simulink model "simulinkProject"  (R2023a)
settings: Solver=ode4  StartTime=0.0  StopTime=20  FixedStep=System.Ts  RelTol=1e-3
values from neighbouring files (symbols this model uses):
  b_end = 0.5*(K_end * (Lift.m + Tilt.m + Cylinder_3.m + Extension_2.m + Extension_1.m + Cylinder_4.m))^0.5    [project.m]
  b_end_1 = 0.5*(K_end_1 * (Lift.m + Pillar.m + Cylinder.m + Tilt.m + Cylinder_4.m + Cylinder_3.m + Extension_1.m + Extension_2.m))^0.5    [project.m]
  b_end_3 = 0.5*(K_end_3 * (Tilt.m + Extension_2.m + Extension_1.m + Cylinder_4.m))^0.5    [project.m]
  b_end_4 = 0.5*(K_end_4 * (Extension_2.m + Extension_1.m))^0.5    [project.m]
  K_end = p_max / delta_x    [project.m]
  K_end_1 = p_max_1 / delta_x_1    [project.m]
  K_end_3 = p_max_3 / delta_x_3    [project.m]
  K_end_4 = p_max_4 / delta_x_4    [project.m]
  Offset = 0.92    [project.m]
  Offset_1 = 0.72    [project.m]
  Offset_4 = 2.640    (= 2.64)    [project.m]
undefined symbols (not defined in the file or in its folder): Cylinder, Cylinder_1, Cylinder_3, Cylinder_4, Extension_1, fabs, Fourbar_1, Fourbar_2, Lift, Pillar, Pinion, Piston, Piston_3, Piston_4, sgn, System, System_1, System_3, System_4, Tilt, Valve, Valve_1, Valve_3, Valve_4, X, Y, Z
libraries: sm_lib x71, nesl_utility x27, TcTargetLib x1
(part 1 of 4)
settings Model: Creator=aless  LastModifiedBy=aless
settings OptimizationCC: DefaultParameterBehavior=Inlined  LocalBlockOutputs=off
settings RTWCC: Description=TwinCAT GRT Target  SystemTargetFile=TwinCatGrt.tlc  GenCodeOnly=on  GenerateMakefile=off  TemplateMakefile=tcgrt_msbuild.tmf  TargetLang=C++
settings STFCustomTargetCC: TargetLangStandard=C++11 (ISO)  CombineOutputUpdateFcns=on  CodeInterfacePackaging=Reusable function  CPPClassGenCompliant=on  GRTInterface=off  GenerateAllocFcn=on  UseToolchainInfoCompliant=off  SystemTargetFile=TwinCatGrt.tlc
settings GRTTargetCC: TargetLangStandard=C++11 (ISO)  ParMdlRefBuildCompliant=off  CompOptLevelCompliant=off  MatFileLogging=off  CodeInterfacePackaging=Reusable function  GenerateAllocFcn=on  UseToolchainInfoCompliant=off  ExtModeMexFile=TcExtModeClient

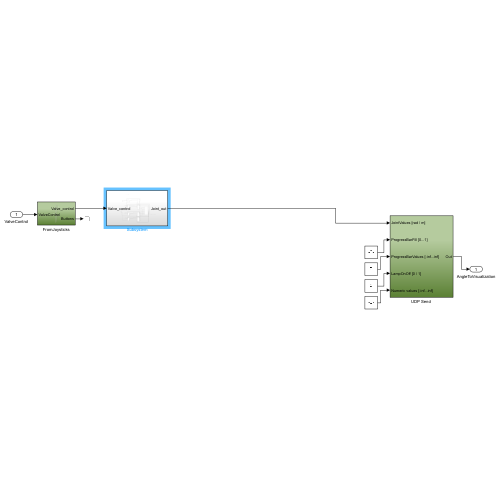
[thumbnail: Simulink's stored preview of the top-level diagram]
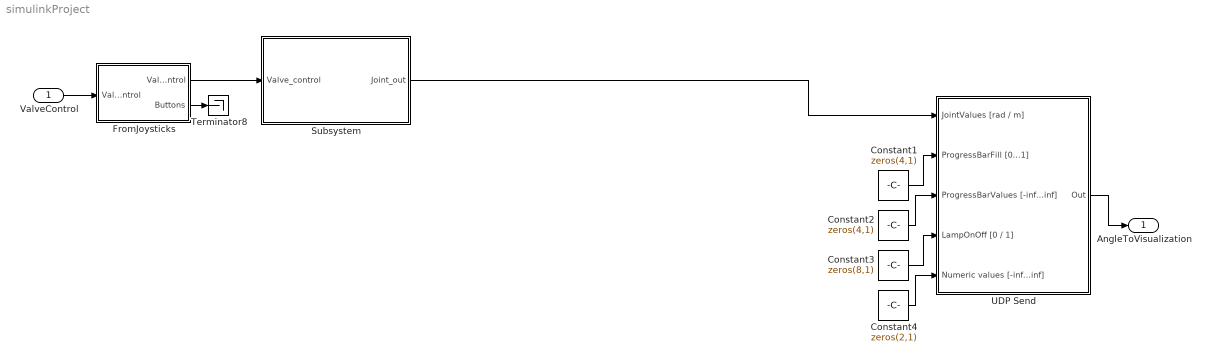
== system simulinkProject ==
  ValveControl : Inport  OutDataTypeStr=double  PortDimensions=19
  Constant1 : Constant  Value=zeros(4,1)
  Constant2 : Constant  Value=zeros(4,1)
  Constant3 : Constant  Value=zeros(8,1)
  Constant4 : Constant  Value=zeros(2,1)
  FromJoysticks : Subsystem
  Subsystem : Subsystem
  Terminator8 : Terminator
  "UDP Send " : Subsystem
  AngleToVisualization : Outport  OutDataTypeStr=single  PortDimensions=22
  wires:
  FromJoysticks/2(Buttons) -> Terminator8/1
  FromJoysticks/1(Valve_control) -> Subsystem/1(Valve_control)
  ValveControl/1 -> FromJoysticks/1(ValveControl)
  "UDP Send "/1(Out) -> AngleToVisualization/1
  Constant2/1 -> "UDP Send "/3(ProgressBarValues [-inf...inf])
  Subsystem/1(Joint_out) -> "UDP Send "/1(JointValues [rad / m])
  Constant1/1 -> "UDP Send "/2(ProgressBarFill [0...1])
  Constant3/1 -> "UDP Send "/4(LampOnOff [0 / 1])
  Constant4/1 -> "UDP Send "/5(Numeric values [-inf...inf])

== system simulinkProject/FromJoysticks ==
  ValveControl : Inport  OutDataTypeStr=double  PortDimensions=19
  Demux : Demux  Outputs=19
  Mux : Mux
  Mux1 : Mux  Inputs=15
  Valve_control : Outport
  Buttons : Outport  Port=2
  wires:
  ValveControl/1 -> Demux/1
  Demux/13 -> Mux1/9
  Demux/15 -> Mux1/11
  Demux/12 -> Mux1/8
  Demux/3 -> Mux/3
  Demux/11 -> Mux1/7
  Demux/16 -> Mux1/12
  Demux/14 -> Mux1/10
  Mux/1 -> Valve_control/1
  Demux/1 -> Mux/1
  Demux/9 -> Mux1/5
  Mux1/1 -> Buttons/1
  Demux/4 -> Mux/4
  Demux/6 -> Mux1/2
  Demux/2 -> Mux/2
  Demux/7 -> Mux1/3
  Demux/10 -> Mux1/6
  Demux/5 -> Mux1/1
  Demux/8 -> Mux1/4
  Demux/17 -> Mux1/13
  Demux/18 -> Mux1/14
  Demux/19 -> Mux1/15

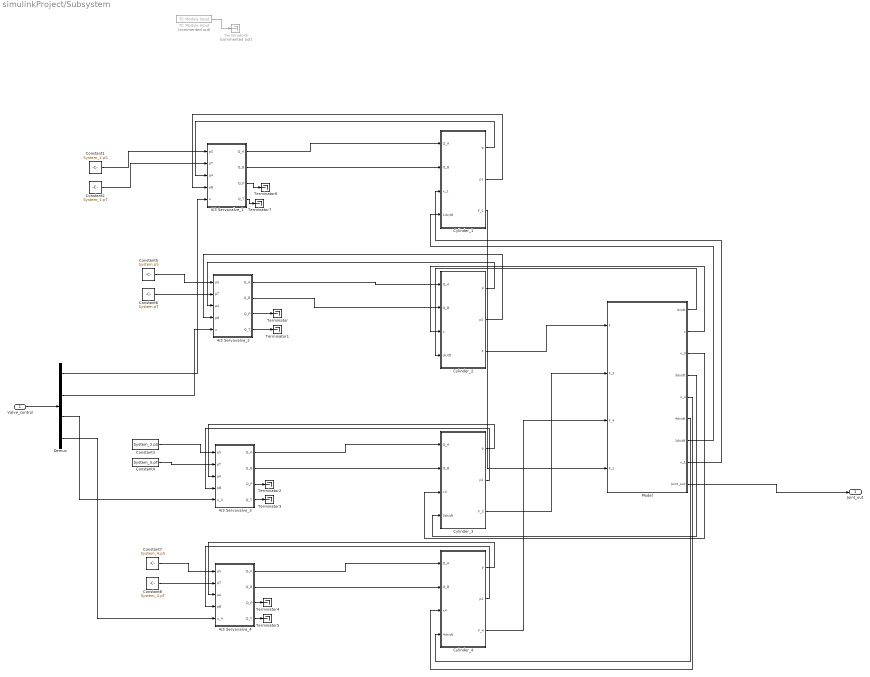
== system simulinkProject/Subsystem ==
  Valve_control : Inport
  4/3 Servovalve_1 : Subsystem  mask(Hydraulic){QN=Valve_1.QN, dpN=Valve_1.dpN, ptr=Valve_1.ptr}
      mask prompts: QN "Nominal flow [m^3/s] :"; dpN "Nominal pressure difference per notch [Pa] :"; ptr "Transition Pressure [Pa] :"
  4/3 Servovalve_2 : Subsystem  mask(Hydraulic){QN=Valve.QN, dpN=Valve.dpN, ptr=Valve.ptr}
      mask prompts: QN "Nominal flow [m^3/s] :"; dpN "Nominal pressure difference per notch [Pa] :"; ptr "Transition Pressure [Pa] :"
  4/3 Servovalve_3 : Subsystem  mask(Hydraulic){QN=Valve_3.QN, dpN=Valve_3.dpN, ptr=Valve_3.ptr}
      mask prompts: QN "Nominal flow [m^3/s] :"; dpN "Nominal pressure difference per notch [Pa] :"; ptr "Transition Pressure [Pa] :"
  4/3 Servovalve_4 : Subsystem  mask(Hydraulic){QN=Valve_4.QN, dpN=Valve_4.dpN, ptr=Valve_4.ptr}
      mask prompts: QN "Nominal flow [m^3/s] :"; dpN "Nominal pressure difference per notch [Pa] :"; ptr "Transition Pressure [Pa] :"
  Constant1 : Constant  Value=System_1.pS
  Constant2 : Constant  Value=System_1.pT
  Constant3 : Constant  Value=System_3.pS
  Constant4 : Constant  Value=System_3.pT
  Constant5 : Constant  Value=System.pS
  Constant6 : Constant  Value=System.pT
  Constant7 : Constant  Value=System_4.pS
  Constant8 : Constant  Value=System_4.pT
  Cylinder_1 : Subsystem
  Cylinder_2 : Subsystem
  Cylinder_3 : Subsystem
  Cylinder_4 : Subsystem
  Demux : Demux
  Model : Subsystem
  TC Module Input : TcTargetLib/TC Module Input  Commented=on  PortDataType=double  PortDim=1  Value=0  SampleTime=-1  CodeGenConnectType=DataArea (InputDst)  DataTypeOverride=off
  Terminator{,1..7} (8 alike) : Terminator
  Terminator8 : Terminator  Commented=on
  Joint_out : Outport
  wires:
  Cylinder_1/3(F_1) -> Model/4(F_1)
  Cylinder_2/1(p) -> 4/3 Servovalve_2/3(pA)
  Model/2(x) -> Cylinder_2/3(x)
  Constant7/1 -> 4/3 Servovalve_4/1(pS)
  Model/8(x_1) -> Cylinder_1/3(x_1)
  4/3 Servovalve_2/2(Q_B) -> Cylinder_2/2(Q_B)
  4/3 Servovalve_1/3(Q_P) -> Terminator6/1
  4/3 Servovalve_2/3(Q_P) -> Terminator/1
  4/3 Servovalve_4/1(Q_A) -> Cylinder_4/1(Q_A)
  Cylinder_4/2(p1) -> 4/3 Servovalve_4/4(pB)
  Cylinder_2/3(F) -> Model/1(F)
  4/3 Servovalve_2/4(Q_T) -> Terminator1/1
  Model/6(4dx/dt) -> Cylinder_4/4(4dx/dt)
  4/3 Servovalve_3/4(Q_T) -> Terminator3/1
  Cylinder_3/2(p1) -> 4/3 Servovalve_3/4(pB)
  Cylinder_4/3(F_4) -> Model/3(F_4)
  Model/5(x_4) -> Cylinder_4/3(x4)
  4/3 Servovalve_3/1(Q_A) -> Cylinder_3/1(Q_A)
  Demux/1 -> 4/3 Servovalve_1/5(u)
  Cylinder_3/3(F_3) -> Model/2(F_3)
  Constant2/1 -> 4/3 Servovalve_1/2(pT)
  Constant3/1 -> 4/3 Servovalve_3/1(pS)
  4/3 Servovalve_2/1(Q_A) -> Cylinder_2/1(Q_A)
  Model/9(Joint_out) -> Joint_out/1
  Cylinder_2/2(p1) -> 4/3 Servovalve_2/4(pB)
  4/3 Servovalve_3/2(Q_B) -> Cylinder_3/2(Q_B)
  Model/3(x_3) -> Cylinder_3/3(x3)
  Cylinder_3/1(p) -> 4/3 Servovalve_3/3(pA)
  4/3 Servovalve_4/2(Q_B) -> Cylinder_4/2(Q_B)
  Model/1(dx/dt) -> Cylinder_2/4(dx/dt)
  4/3 Servovalve_4/4(Q_T) -> Terminator5/1
  Constant4/1 -> 4/3 Servovalve_3/2(pT)
  Model/4(3dx/dt) -> Cylinder_3/4(3dx/dt)
  Constant6/1 -> 4/3 Servovalve_2/2(pT)
  4/3 Servovalve_1/1(Q_A) -> Cylinder_1/1(Q_A)
  Cylinder_4/1(p) -> 4/3 Servovalve_4/3(pA)
  Constant1/1 -> 4/3 Servovalve_1/1(pS)
  4/3 Servovalve_4/3(Q_P) -> Terminator4/1
  4/3 Servovalve_1/4(Q_T) -> Terminator7/1
  Constant5/1 -> 4/3 Servovalve_2/1(pS)
  Demux/2 -> 4/3 Servovalve_2/5(u)
  Constant8/1 -> 4/3 Servovalve_4/2(pT)
  4/3 Servovalve_1/2(Q_B) -> Cylinder_1/2(Q_B)
  4/3 Servovalve_3/3(Q_P) -> Terminator2/1
  Valve_control/1 -> Demux/1
  Cylinder_1/1(p) -> 4/3 Servovalve_1/3(pA)
  Model/7(1dx/dt) -> Cylinder_1/4(1dx/dt)
  Cylinder_1/2(p1) -> 4/3 Servovalve_1/4(pB)
  Demux/4 -> 4/3 Servovalve_4/5(u_4)
  TC Module Input/1 -> Terminator8/1
  Demux/3 -> 4/3 Servovalve_3/5(u_3)

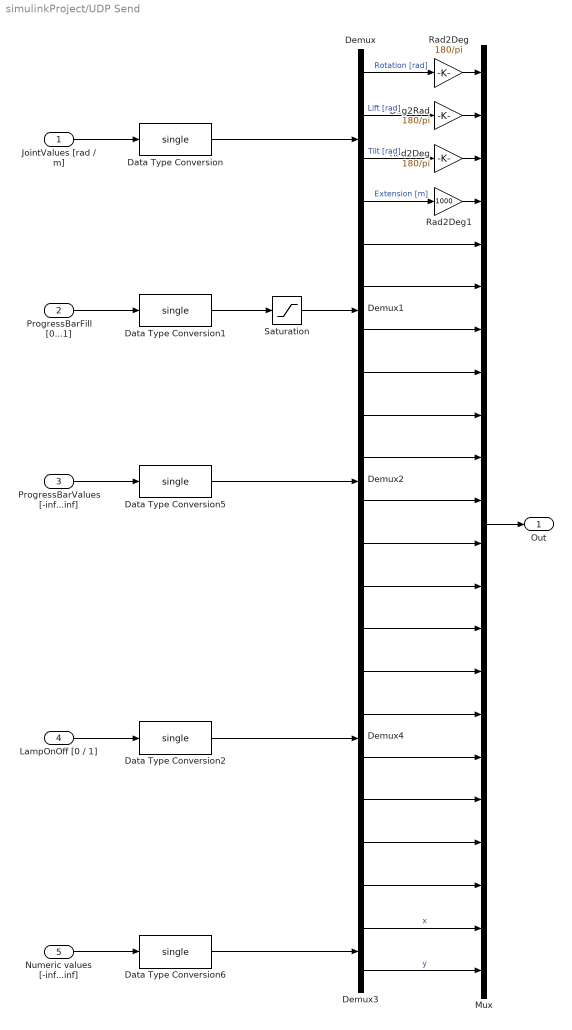
== system simulinkProject/UDP Send  ==
  JointValues [rad / m] : Inport
  ProgressBarFill [0...1] : Inport  Port=2
  ProgressBarValues [-inf...inf] : Inport  Port=3
  LampOnOff [0 / 1] : Inport  Port=4
  Numeric values [-inf...inf] : Inport  Port=5
  Data Type Conversion{,1..2,5..6} (5 alike) : DataTypeConversion  OutDataTypeStr=single  SaturateOnIntegerOverflow=off  RndMeth=Floor
  "Deg2Rad " : Gain  Gain=180/pi
  Demux : Demux
  Demux1 : Demux
  Demux2 : Demux
  Demux3 : Demux  Outputs=2
  Demux4 : Demux  Outputs=8
  Mux : Mux  Inputs=22
  Rad2Deg : Gain  Gain=180/pi
  "Rad2Deg " : Gain  Gain=180/pi
  Rad2Deg1 : Gain  Gain=1000
  Saturation : Saturate  UpperLimit=1  LowerLimit=0
  Out : Outport  OutDataTypeStr=single  PortDimensions=22
  wires:
  JointValues [rad / m]/1 -> Data Type Conversion/1
  Demux/4 -> Rad2Deg1/1  "Extension [m]"
  Demux/2 -> "Deg2Rad "/1  "Lift [rad]"
  Demux/3 -> Rad2Deg/1  "Tilt [rad]"
  Demux/1 -> "Rad2Deg "/1  "Rotation [rad]"
  "Rad2Deg "/1 -> Mux/1
  "Deg2Rad "/1 -> Mux/2
  Rad2Deg/1 -> Mux/3
  Data Type Conversion/1 -> Demux/1
  Demux1/1 -> Mux/5
  Demux1/2 -> Mux/6
  Demux1/3 -> Mux/7
  Demux1/4 -> Mux/8
  Demux2/1 -> Mux/9
  Demux2/2 -> Mux/10
  Demux2/3 -> Mux/11
  Demux2/4 -> Mux/12
  Data Type Conversion1/1 -> Saturation/1
  Data Type Conversion5/1 -> Demux2/1
  Demux4/1 -> Mux/13
  Demux4/2 -> Mux/14
  Demux4/3 -> Mux/15
  Demux4/4 -> Mux/16
  Demux4/5 -> Mux/17
  Demux4/6 -> Mux/18
  Demux4/7 -> Mux/19
  Demux4/8 -> Mux/20
  Demux3/1 -> Mux/21  "x"
  Demux3/2 -> Mux/22  "y"
  LampOnOff [0 / 1]/1 -> Data Type Conversion2/1
  Data Type Conversion2/1 -> Demux4/1
  Saturation/1 -> Demux1/1
  ProgressBarFill [0...1]/1 -> Data Type Conversion1/1
  ProgressBarValues [-inf...inf]/1 -> Data Type Conversion5/1
  Numeric values [-inf...inf]/1 -> Data Type Conversion6/1
  Data Type Conversion6/1 -> Demux3/1
  Mux/1 -> Out/1
  Rad2Deg1/1 -> Mux/4

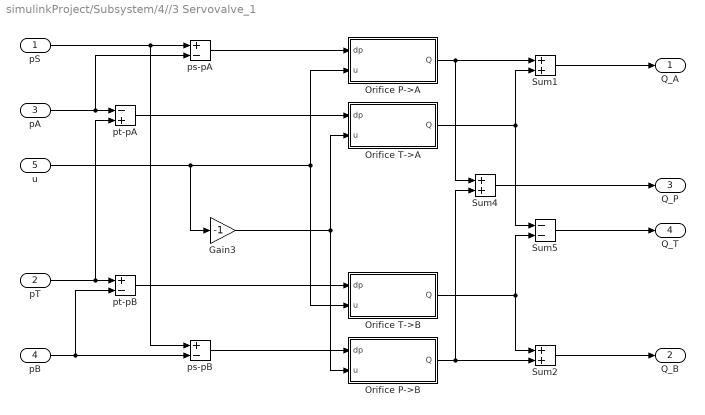
== system simulinkProject/Subsystem/4//3 Servovalve_1 ==
  pS : Inport
  pT : Inport  Port=2
  pA : Inport  Port=3
  pB : Inport  Port=4
  u : Inport  Port=5
  Gain3 : Gain  Gain=-1  SaturateOnIntegerOverflow=on  OutDataTypeStr=Inherit: Same as input  ParamDataTypeStr=Inherit: Same as input
  Orifice P->A : Subsystem  mask(Hydraulic){QN=QN, AN=1, DPN=dpN, ptr=ptr}
      mask prompts: QN "Nominal Flow [m^3/s] :"; AN "Nominal opening [ 0...1 ] :"; DPN "Nominal Pressure Difference [Pa] :"; ptr "Transition Pressure [Pa] :"
      mask help:
      | Implements numerically robust turbulent flow
      | equation. Polynomial flow equation is used
      | when abs(dp) < Transition Pressure.
      mask init:
      | K = QN/(AN*sqrt(DPN));
      mask Help: eval('hydlibdoc(''orificedoc'')')
  Orifice P->B : Subsystem  mask(Hydraulic){QN=QN, AN=1, DPN=dpN, ptr=ptr}
      mask prompts: QN "Nominal Flow [m^3/s] :"; AN "Nominal opening [ 0...1 ] :"; DPN "Nominal Pressure Difference [Pa] :"; ptr "Transition Pressure [Pa] :"
      mask help:
      | Implements numerically robust turbulent flow
      | equation. Polynomial flow equation is used
      | when abs(dp) < Transition Pressure.
      mask init:
      | K = QN/(AN*sqrt(DPN));
      mask Help: eval('hydlibdoc(''orificedoc'')')
  Orifice T->A : Subsystem  mask(Hydraulic){QN=QN, AN=1, DPN=dpN, ptr=ptr}
      mask prompts: QN "Nominal Flow [m^3/s] :"; AN "Nominal opening [ 0...1 ] :"; DPN "Nominal Pressure Difference [Pa] :"; ptr "Transition Pressure [Pa] :"
      mask help:
      | Implements numerically robust turbulent flow
      | equation. Polynomial flow equation is used
      | when abs(dp) < Transition Pressure.
      mask init:
      | K = QN/(AN*sqrt(DPN));
      mask Help: eval('hydlibdoc(''orificedoc'')')
  Orifice T->B : Subsystem  mask(Hydraulic){QN=QN, AN=1, DPN=dpN, ptr=ptr}
      mask prompts: QN "Nominal Flow [m^3/s] :"; AN "Nominal opening [ 0...1 ] :"; DPN "Nominal Pressure Difference [Pa] :"; ptr "Transition Pressure [Pa] :"
      mask help:
      | Implements numerically robust turbulent flow
      | equation. Polynomial flow equation is used
      | when abs(dp) < Transition Pressure.
      mask init:
      | K = QN/(AN*sqrt(DPN));
      mask Help: eval('hydlibdoc(''orificedoc'')')
  Sum1 : Sum  InputSameDT=on  SaturateOnIntegerOverflow=on  OutDataTypeStr=Inherit: Same as first input
  Sum2 : Sum  InputSameDT=on  SaturateOnIntegerOverflow=on  OutDataTypeStr=Inherit: Same as first input
  Sum4 : Sum  InputSameDT=on  SaturateOnIntegerOverflow=on  OutDataTypeStr=Inherit: Same as first input
  Sum5 : Sum  Inputs=--  InputSameDT=on  SaturateOnIntegerOverflow=on  OutDataTypeStr=Inherit: Same as first input
  ps-pA : Sum  Inputs=+-  InputSameDT=on  SaturateOnIntegerOverflow=on  OutDataTypeStr=Inherit: Same as first input
  ps-pB : Sum  Inputs=+-  InputSameDT=on  SaturateOnIntegerOverflow=on  OutDataTypeStr=Inherit: Same as first input
  pt-pA : Sum  Inputs=-+  InputSameDT=on  SaturateOnIntegerOverflow=on  OutDataTypeStr=Inherit: Same as first input
  pt-pB : Sum  Inputs=+-  InputSameDT=on  SaturateOnIntegerOverflow=on  OutDataTypeStr=Inherit: Same as first input
  Q_A : Outport  VectorParamsAs1DForOutWhenUnconnected=off
  Q_B : Outport  Port=2  VectorParamsAs1DForOutWhenUnconnected=off
  Q_P : Outport  Port=3  VectorParamsAs1DForOutWhenUnconnected=off
  Q_T : Outport  Port=4  VectorParamsAs1DForOutWhenUnconnected=off
  wires:
  Gain3/1 -> Orifice P->B/2(u), Orifice T->A/2(u)
  pt-pB/1 -> Orifice T->B/1(dp)
  ps-pB/1 -> Orifice P->B/1(dp)
  ps-pA/1 -> Orifice P->A/1(dp)
  pt-pA/1 -> Orifice T->A/1(dp)
  Sum5/1 -> Q_T/1
  Sum4/1 -> Q_P/1
  Orifice P->A/1(Q) -> Sum4/1, Sum1/1
  Orifice P->B/1(Q) -> Sum4/2, Sum2/2
  u/1 -> Orifice T->B/2(u), Orifice P->A/2(u), Gain3/1
  pB/1 -> pt-pB/2, ps-pB/2
  Orifice T->B/1(Q) -> Sum2/1, Sum5/2
  Sum2/1 -> Q_B/1
  pT/1 -> pt-pA/2, pt-pB/1
  pA/1 -> ps-pA/2, pt-pA/1
  pS/1 -> ps-pA/1, ps-pB/1
  Orifice T->A/1(Q) -> Sum1/2, Sum5/1
  Sum1/1 -> Q_A/1

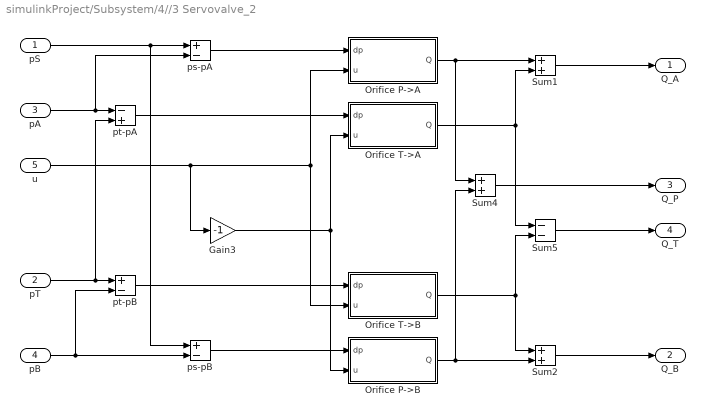
== system simulinkProject/Subsystem/4//3 Servovalve_2 ==
  pS : Inport
  pT : Inport  Port=2
  pA : Inport  Port=3
  pB : Inport  Port=4
  u : Inport  Port=5
  Gain3 : Gain  Gain=-1  SaturateOnIntegerOverflow=on  OutDataTypeStr=Inherit: Same as input  ParamDataTypeStr=Inherit: Same as input
  Orifice P->A : Subsystem  mask(Hydraulic){QN=QN, AN=1, DPN=dpN, ptr=ptr}
      mask prompts: QN "Nominal Flow [m^3/s] :"; AN "Nominal opening [ 0...1 ] :"; DPN "Nominal Pressure Difference [Pa] :"; ptr "Transition Pressure [Pa] :"
      mask help:
      | Implements numerically robust turbulent flow
      | equation. Polynomial flow equation is used
      | when abs(dp) < Transition Pressure.
      mask init:
      | K = QN/(AN*sqrt(DPN));
      mask Help: eval('hydlibdoc(''orificedoc'')')
  Orifice P->B : Subsystem  mask(Hydraulic){QN=QN, AN=1, DPN=dpN, ptr=ptr}
      mask prompts: QN "Nominal Flow [m^3/s] :"; AN "Nominal opening [ 0...1 ] :"; DPN "Nominal Pressure Difference [Pa] :"; ptr "Transition Pressure [Pa] :"
      mask help:
      | Implements numerically robust turbulent flow
      | equation. Polynomial flow equation is used
      | when abs(dp) < Transition Pressure.
      mask init:
      | K = QN/(AN*sqrt(DPN));
      mask Help: eval('hydlibdoc(''orificedoc'')')
  Orifice T->A : Subsystem  mask(Hydraulic){QN=QN, AN=1, DPN=dpN, ptr=ptr}
      mask prompts: QN "Nominal Flow [m^3/s] :"; AN "Nominal opening [ 0...1 ] :"; DPN "Nominal Pressure Difference [Pa] :"; ptr "Transition Pressure [Pa] :"
      mask help:
      | Implements numerically robust turbulent flow
      | equation. Polynomial flow equation is used
      | when abs(dp) < Transition Pressure.
      mask init:
      | K = QN/(AN*sqrt(DPN));
      mask Help: eval('hydlibdoc(''orificedoc'')')
  Orifice T->B : Subsystem  mask(Hydraulic){QN=QN, AN=1, DPN=dpN, ptr=ptr}
      mask prompts: QN "Nominal Flow [m^3/s] :"; AN "Nominal opening [ 0...1 ] :"; DPN "Nominal Pressure Difference [Pa] :"; ptr "Transition Pressure [Pa] :"
      mask help:
      | Implements numerically robust turbulent flow
      | equation. Polynomial flow equation is used
      | when abs(dp) < Transition Pressure.
      mask init:
      | K = QN/(AN*sqrt(DPN));
      mask Help: eval('hydlibdoc(''orificedoc'')')
  Sum1 : Sum  InputSameDT=on  SaturateOnIntegerOverflow=on  OutDataTypeStr=Inherit: Same as first input
  Sum2 : Sum  InputSameDT=on  SaturateOnIntegerOverflow=on  OutDataTypeStr=Inherit: Same as first input
  Sum4 : Sum  InputSameDT=on  SaturateOnIntegerOverflow=on  OutDataTypeStr=Inherit: Same as first input
  Sum5 : Sum  Inputs=--  InputSameDT=on  SaturateOnIntegerOverflow=on  OutDataTypeStr=Inherit: Same as first input
  ps-pA : Sum  Inputs=+-  InputSameDT=on  SaturateOnIntegerOverflow=on  OutDataTypeStr=Inherit: Same as first input
  ps-pB : Sum  Inputs=+-  InputSameDT=on  SaturateOnIntegerOverflow=on  OutDataTypeStr=Inherit: Same as first input
  pt-pA : Sum  Inputs=-+  InputSameDT=on  SaturateOnIntegerOverflow=on  OutDataTypeStr=Inherit: Same as first input
  pt-pB : Sum  Inputs=+-  InputSameDT=on  SaturateOnIntegerOverflow=on  OutDataTypeStr=Inherit: Same as first input
  Q_A : Outport  VectorParamsAs1DForOutWhenUnconnected=off
  Q_B : Outport  Port=2  VectorParamsAs1DForOutWhenUnconnected=off
  Q_P : Outport  Port=3  VectorParamsAs1DForOutWhenUnconnected=off
  Q_T : Outport  Port=4  VectorParamsAs1DForOutWhenUnconnected=off
  wires:
  Gain3/1 -> Orifice P->B/2(u), Orifice T->A/2(u)
  pt-pB/1 -> Orifice T->B/1(dp)
  ps-pB/1 -> Orifice P->B/1(dp)
  ps-pA/1 -> Orifice P->A/1(dp)
  pt-pA/1 -> Orifice T->A/1(dp)
  Sum5/1 -> Q_T/1
  Sum4/1 -> Q_P/1
  Orifice P->A/1(Q) -> Sum4/1, Sum1/1
  Orifice P->B/1(Q) -> Sum4/2, Sum2/2
  u/1 -> Orifice T->B/2(u), Orifice P->A/2(u), Gain3/1
  pB/1 -> pt-pB/2, ps-pB/2
  Orifice T->B/1(Q) -> Sum2/1, Sum5/2
  Sum2/1 -> Q_B/1
  pT/1 -> pt-pA/2, pt-pB/1
  pA/1 -> ps-pA/2, pt-pA/1
  pS/1 -> ps-pA/1, ps-pB/1
  Orifice T->A/1(Q) -> Sum1/2, Sum5/1
  Sum1/1 -> Q_A/1

== system simulinkProject/Subsystem/4//3 Servovalve_3 ==
  pS : Inport
  pT : Inport  Port=2
  pA : Inport  Port=3
  pB : Inport  Port=4
  u_3 : Inport  Port=5
  Gain3 : Gain  Gain=-1  SaturateOnIntegerOverflow=on  OutDataTypeStr=Inherit: Same as input  ParamDataTypeStr=Inherit: Same as input
  Orifice P->A : Subsystem  mask(Hydraulic){QN=QN, AN=1, DPN=dpN, ptr=ptr}
      mask prompts: QN "Nominal Flow [m^3/s] :"; AN "Nominal opening [ 0...1 ] :"; DPN "Nominal Pressure Difference [Pa] :"; ptr "Transition Pressure [Pa] :"
      mask help:
      | Implements numerically robust turbulent flow
      | equation. Polynomial flow equation is used
      | when abs(dp) < Transition Pressure.
      mask init:
      | K = QN/(AN*sqrt(DPN));
      mask Help: eval('hydlibdoc(''orificedoc'')')
  Orifice P->B : Subsystem  mask(Hydraulic){QN=QN, AN=1, DPN=dpN, ptr=ptr}
      mask prompts: QN "Nominal Flow [m^3/s] :"; AN "Nominal opening [ 0...1 ] :"; DPN "Nominal Pressure Difference [Pa] :"; ptr "Transition Pressure [Pa] :"
      mask help:
      | Implements numerically robust turbulent flow
      | equation. Polynomial flow equation is used
      | when abs(dp) < Transition Pressure.
      mask init:
      | K = QN/(AN*sqrt(DPN));
      mask Help: eval('hydlibdoc(''orificedoc'')')
  Orifice T->A : Subsystem  mask(Hydraulic){QN=QN, AN=1, DPN=dpN, ptr=ptr}
      mask prompts: QN "Nominal Flow [m^3/s] :"; AN "Nominal opening [ 0...1 ] :"; DPN "Nominal Pressure Difference [Pa] :"; ptr "Transition Pressure [Pa] :"
      mask help:
      | Implements numerically robust turbulent flow
      | equation. Polynomial flow equation is used
      | when abs(dp) < Transition Pressure.
      mask init:
      | K = QN/(AN*sqrt(DPN));
      mask Help: eval('hydlibdoc(''orificedoc'')')
  Orifice T->B : Subsystem  mask(Hydraulic){QN=QN, AN=1, DPN=dpN, ptr=ptr}
      mask prompts: QN "Nominal Flow [m^3/s] :"; AN "Nominal opening [ 0...1 ] :"; DPN "Nominal Pressure Difference [Pa] :"; ptr "Transition Pressure [Pa] :"
      mask help:
      | Implements numerically robust turbulent flow
      | equation. Polynomial flow equation is used
      | when abs(dp) < Transition Pressure.
      mask init:
      | K = QN/(AN*sqrt(DPN));
      mask Help: eval('hydlibdoc(''orificedoc'')')
  Sum1 : Sum  InputSameDT=on  SaturateOnIntegerOverflow=on  OutDataTypeStr=Inherit: Same as first input
  Sum2 : Sum  InputSameDT=on  SaturateOnIntegerOverflow=on  OutDataTypeStr=Inherit: Same as first input
  Sum4 : Sum  InputSameDT=on  SaturateOnIntegerOverflow=on  OutDataTypeStr=Inherit: Same as first input
  Sum5 : Sum  Inputs=--  InputSameDT=on  SaturateOnIntegerOverflow=on  OutDataTypeStr=Inherit: Same as first input
  ps-pA : Sum  Inputs=+-  InputSameDT=on  SaturateOnIntegerOverflow=on  OutDataTypeStr=Inherit: Same as first input
  ps-pB : Sum  Inputs=+-  InputSameDT=on  SaturateOnIntegerOverflow=on  OutDataTypeStr=Inherit: Same as first input
  pt-pA : Sum  Inputs=-+  InputSameDT=on  SaturateOnIntegerOverflow=on  OutDataTypeStr=Inherit: Same as first input
  pt-pB : Sum  Inputs=+-  InputSameDT=on  SaturateOnIntegerOverflow=on  OutDataTypeStr=Inherit: Same as first input
  Q_A : Outport  VectorParamsAs1DForOutWhenUnconnected=off
  Q_B : Outport  Port=2  VectorParamsAs1DForOutWhenUnconnected=off
  Q_P : Outport  Port=3  VectorParamsAs1DForOutWhenUnconnected=off
  Q_T : Outport  Port=4  VectorParamsAs1DForOutWhenUnconnected=off
  wires:
  Gain3/1 -> Orifice P->B/2(u), Orifice T->A/2(u)
  pt-pB/1 -> Orifice T->B/1(dp)
  ps-pB/1 -> Orifice P->B/1(dp)
  ps-pA/1 -> Orifice P->A/1(dp)
  pt-pA/1 -> Orifice T->A/1(dp)
  Sum5/1 -> Q_T/1
  Sum4/1 -> Q_P/1
  Orifice P->A/1(Q) -> Sum4/1, Sum1/1
  Orifice P->B/1(Q) -> Sum4/2, Sum2/2
  u_3/1 -> Orifice T->B/2(u), Orifice P->A/2(u), Gain3/1
  pB/1 -> pt-pB/2, ps-pB/2
  Orifice T->B/1(Q) -> Sum2/1, Sum5/2
  Sum2/1 -> Q_B/1
  pT/1 -> pt-pA/2, pt-pB/1
  pA/1 -> ps-pA/2, pt-pA/1
  pS/1 -> ps-pA/1, ps-pB/1
  Orifice T->A/1(Q) -> Sum1/2, Sum5/1
  Sum1/1 -> Q_A/1

== system simulinkProject/Subsystem/4//3 Servovalve_4 ==
  pS : Inport
  pT : Inport  Port=2
  pA : Inport  Port=3
  pB : Inport  Port=4
  u_4 : Inport  Port=5
  Gain3 : Gain  Gain=-1  SaturateOnIntegerOverflow=on  OutDataTypeStr=Inherit: Same as input  ParamDataTypeStr=Inherit: Same as input
  Orifice P->A : Subsystem  mask(Hydraulic){QN=QN, AN=1, DPN=dpN, ptr=ptr}
      mask prompts: QN "Nominal Flow [m^3/s] :"; AN "Nominal opening [ 0...1 ] :"; DPN "Nominal Pressure Difference [Pa] :"; ptr "Transition Pressure [Pa] :"
      mask help:
      | Implements numerically robust turbulent flow
      | equation. Polynomial flow equation is used
      | when abs(dp) < Transition Pressure.
      mask init:
      | K = QN/(AN*sqrt(DPN));
      mask Help: eval('hydlibdoc(''orificedoc'')')
  Orifice P->B : Subsystem  mask(Hydraulic){QN=QN, AN=1, DPN=dpN, ptr=ptr}
      mask prompts: QN "Nominal Flow [m^3/s] :"; AN "Nominal opening [ 0...1 ] :"; DPN "Nominal Pressure Difference [Pa] :"; ptr "Transition Pressure [Pa] :"
      mask help:
      | Implements numerically robust turbulent flow
      | equation. Polynomial flow equation is used
      | when abs(dp) < Transition Pressure.
      mask init:
      | K = QN/(AN*sqrt(DPN));
      mask Help: eval('hydlibdoc(''orificedoc'')')
  Orifice T->A : Subsystem  mask(Hydraulic){QN=QN, AN=1, DPN=dpN, ptr=ptr}
      mask prompts: QN "Nominal Flow [m^3/s] :"; AN "Nominal opening [ 0...1 ] :"; DPN "Nominal Pressure Difference [Pa] :"; ptr "Transition Pressure [Pa] :"
      mask help:
      | Implements numerically robust turbulent flow
      | equation. Polynomial flow equation is used
      | when abs(dp) < Transition Pressure.
      mask init:
      | K = QN/(AN*sqrt(DPN));
      mask Help: eval('hydlibdoc(''orificedoc'')')
  Orifice T->B : Subsystem  mask(Hydraulic){QN=QN, AN=1, DPN=dpN, ptr=ptr}
      mask prompts: QN "Nominal Flow [m^3/s] :"; AN "Nominal opening [ 0...1 ] :"; DPN "Nominal Pressure Difference [Pa] :"; ptr "Transition Pressure [Pa] :"
      mask help:
      | Implements numerically robust turbulent flow
      | equation. Polynomial flow equation is used
      | when abs(dp) < Transition Pressure.
      mask init:
      | K = QN/(AN*sqrt(DPN));
      mask Help: eval('hydlibdoc(''orificedoc'')')
  Sum1 : Sum  InputSameDT=on  SaturateOnIntegerOverflow=on  OutDataTypeStr=Inherit: Same as first input
  Sum2 : Sum  InputSameDT=on  SaturateOnIntegerOverflow=on  OutDataTypeStr=Inherit: Same as first input
  Sum4 : Sum  InputSameDT=on  SaturateOnIntegerOverflow=on  OutDataTypeStr=Inherit: Same as first input
  Sum5 : Sum  Inputs=--  InputSameDT=on  SaturateOnIntegerOverflow=on  OutDataTypeStr=Inherit: Same as first input
  ps-pA : Sum  Inputs=+-  InputSameDT=on  SaturateOnIntegerOverflow=on  OutDataTypeStr=Inherit: Same as first input
  ps-pB : Sum  Inputs=+-  InputSameDT=on  SaturateOnIntegerOverflow=on  OutDataTypeStr=Inherit: Same as first input
  pt-pA : Sum  Inputs=-+  InputSameDT=on  SaturateOnIntegerOverflow=on  OutDataTypeStr=Inherit: Same as first input
  pt-pB : Sum  Inputs=+-  InputSameDT=on  SaturateOnIntegerOverflow=on  OutDataTypeStr=Inherit: Same as first input
  Q_A : Outport  VectorParamsAs1DForOutWhenUnconnected=off
  Q_B : Outport  Port=2  VectorParamsAs1DForOutWhenUnconnected=off
  Q_P : Outport  Port=3  VectorParamsAs1DForOutWhenUnconnected=off
  Q_T : Outport  Port=4  VectorParamsAs1DForOutWhenUnconnected=off
  wires:
  Gain3/1 -> Orifice P->B/2(u), Orifice T->A/2(u)
  pt-pB/1 -> Orifice T->B/1(dp)
  ps-pB/1 -> Orifice P->B/1(dp)
  ps-pA/1 -> Orifice P->A/1(dp)
  pt-pA/1 -> Orifice T->A/1(dp)
  Sum5/1 -> Q_T/1
  Sum4/1 -> Q_P/1
  Orifice P->A/1(Q) -> Sum4/1, Sum1/1
  Orifice P->B/1(Q) -> Sum4/2, Sum2/2
  u_4/1 -> Orifice T->B/2(u), Orifice P->A/2(u), Gain3/1
  pB/1 -> pt-pB/2, ps-pB/2
  Orifice T->B/1(Q) -> Sum2/1, Sum5/2
  Sum2/1 -> Q_B/1
  pT/1 -> pt-pA/2, pt-pB/1
  pA/1 -> ps-pA/2, pt-pA/1
  pS/1 -> ps-pA/1, ps-pB/1
  Orifice T->A/1(Q) -> Sum1/2, Sum5/1
  Sum1/1 -> Q_A/1

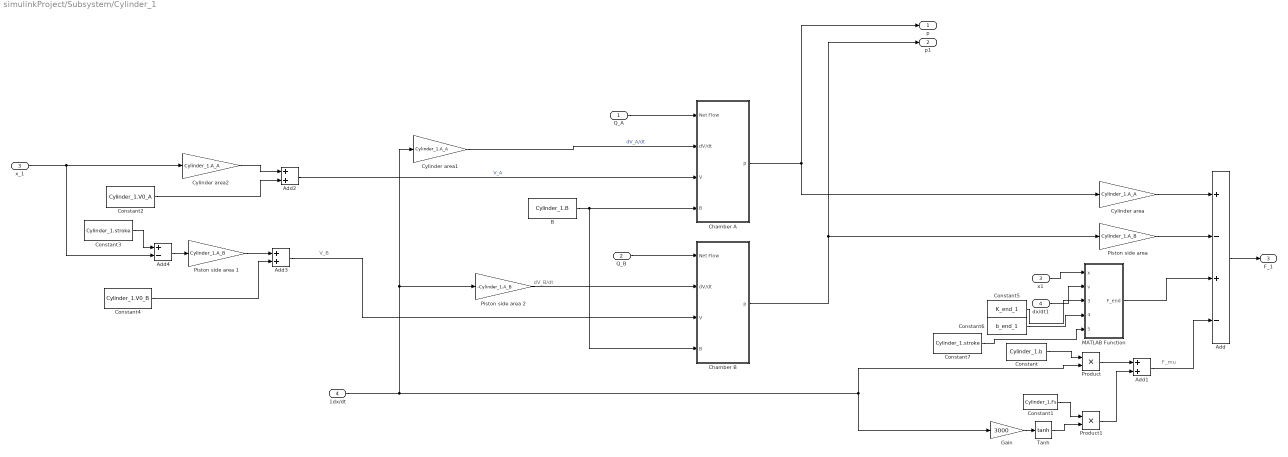
== system simulinkProject/Subsystem/Cylinder_1 ==
  note: dV_B/dt
  note: V_B
  note: F_mu
  Q_A : Inport
  Q_B : Inport  Port=2
  x_1 : Inport  Port=3
  1dx/dt : Inport  Port=4
  Add : Sum  Inputs=+-+-
  Add1 : Sum
  Add2 : Sum
  Add3 : Sum
  Add4 : Sum  Inputs=+-
  B : Constant  Value=Cylinder_1.B
  Chamber A : Subsystem  mask(Hydraulic){pinitial=Cylinder.p0_A}
      mask prompts: pinitial "Initial pressure [Pa] :"
      mask help: Lumped fluid volume. Pressure is limited greater or equal to zero by saturation block corresponding to a rough model of cavitation.
      mask Help: eval('hydlibdoc(''vol_cav_doc'')')
  Chamber B : Subsystem  mask(Hydraulic){pinitial=Cylinder.p0_B}
      mask prompts: pinitial "Initial pressure [Pa] :"
      mask help: Lumped fluid volume. Pressure is limited greater or equal to zero by saturation block corresponding to a rough model of cavitation.
      mask Help: eval('hydlibdoc(''vol_cav_doc'')')
  Constant : Constant  Value=Cylinder_1.b
  Constant1 : Constant  Value=Cylinder_1.Fs
  Constant2 : Constant  Value=Cylinder_1.V0_A
  Constant3 : Constant  Value=Cylinder_1.stroke
  Constant4 : Constant  Value=Cylinder_1.V0_B
  Constant5 : Constant  Value=K_end_1
  Constant6 : Constant  Value=b_end_1
  Constant7 : Constant  Value=Cylinder_1.stroke
  Cylinder area : Gain  Gain=Cylinder_1.A_A
  Cylinder area1 : Gain  Gain=Cylinder_1.A_A
  Cylinder area2 : Gain  Gain=Cylinder_1.A_A
  Gain : Gain  Gain=3000
  MATLAB Function : MATLAB Function  TreatAsAtomicUnit=on
  "Piston side area " : Gain  Gain=Cylinder_1.A_B
  Piston side area 1 : Gain  Gain=Cylinder_1.A_B
  Piston side area 2 : Gain  Gain=-Cylinder_1.A_B
  Product : Product
  Product1 : Product
  Tanh : Trigonometry  Operator=tanh
  dx/dt1 : InportShadow  Port=4
  x1 : InportShadow  Port=3
  p : Outport
  p1 : Outport  Port=2
  F_1 : Outport  Port=3
  wires:
  B/1 -> Chamber B/4(" B"), Chamber A/4(" B")
  Piston side area 2/1 -> Chamber B/2(" dV/dt")
  Constant/1 -> Product/1
  Add3/1 -> Chamber B/3(" V")
  x_1/1 -> Add4/2, Cylinder area2/1
  Chamber B/1(p) -> p1/1, "Piston side area "/1
  Tanh/1 -> Product1/2
  Q_A/1 -> Chamber A/1(Net Flow)
  Gain/1 -> Tanh/1
  Chamber A/1(p) -> p/1, Cylinder area/1
  Constant4/1 -> Add3/2
  Piston side area 1/1 -> Add3/1
  Add/1 -> F_1/1
  Q_B/1 -> Chamber B/1(Net Flow)
  1dx/dt/1 -> Product/2, Gain/1, Cylinder area1/1, Piston side area 2/1
  Constant1/1 -> Product1/1
  Cylinder area2/1 -> Add2/1
  Constant2/1 -> Add2/2
  Product1/1 -> Add1/2
  Add1/1 -> Add/4
  Cylinder area1/1 -> Chamber A/2(" dV/dt")  "dV_A/dt"
  Product/1 -> Add1/1
  "Piston side area "/1 -> Add/2
  Add2/1 -> Chamber A/3(" V")  "V_A"
  Cylinder area/1 -> Add/1
  Add4/1 -> Piston side area 1/1
  Constant3/1 -> Add4/1
  dx/dt1/1 -> MATLAB Function/2(v)
  x1/1 -> MATLAB Function/1(x)
  Constant5/1 -> MATLAB Function/3(K_end_1)
  Constant6/1 -> MATLAB Function/4(b_end_1)
  MATLAB Function/1(F_end) -> Add/3
  Constant7/1 -> MATLAB Function/5(Cylinder_1stroke)

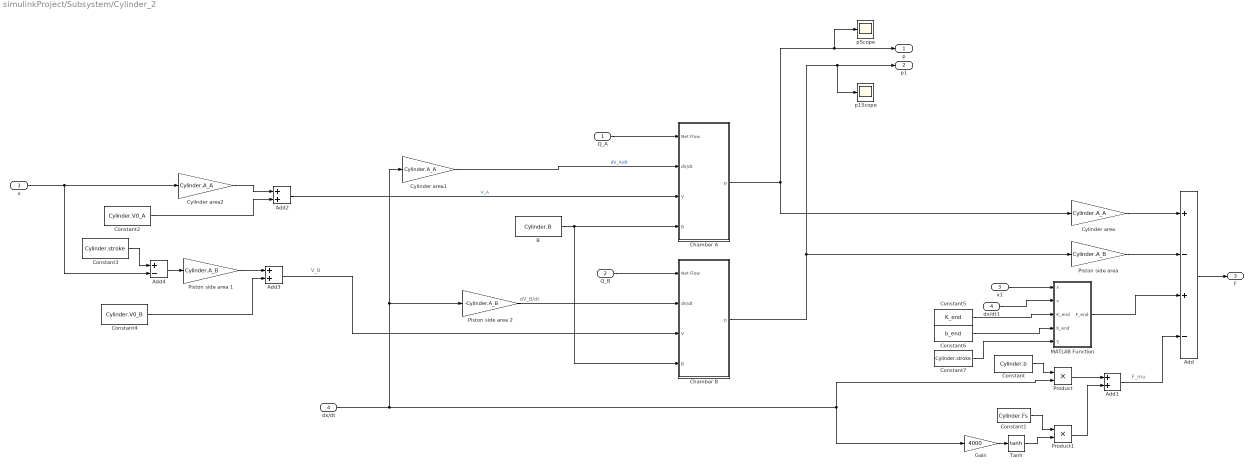
== system simulinkProject/Subsystem/Cylinder_2 ==
  note: dV_B/dt
  note: V_B
  note: F_mu
  Q_A : Inport
  Q_B : Inport  Port=2
  x : Inport  Port=3
  dx/dt : Inport  Port=4
  Add : Sum  Inputs=+-+-
  Add1 : Sum
  Add2 : Sum
  Add3 : Sum
  Add4 : Sum  Inputs=+-
  B : Constant  Value=Cylinder.B
  Chamber A : Subsystem  mask(Hydraulic){pinitial=Cylinder.p0_A}
      mask prompts: pinitial "Initial pressure [Pa] :"
      mask help: Lumped fluid volume. Pressure is limited greater or equal to zero by saturation block corresponding to a rough model of cavitation.
      mask Help: eval('hydlibdoc(''vol_cav_doc'')')
  Chamber B : Subsystem  mask(Hydraulic){pinitial=Cylinder.p0_B}
      mask prompts: pinitial "Initial pressure [Pa] :"
      mask help: Lumped fluid volume. Pressure is limited greater or equal to zero by saturation block corresponding to a rough model of cavitation.
      mask Help: eval('hydlibdoc(''vol_cav_doc'')')
  Constant : Constant  Value=Cylinder.b
  Constant1 : Constant  Value=Cylinder.Fs
  Constant2 : Constant  Value=Cylinder.V0_A
  Constant3 : Constant  Value=Cylinder.stroke
  Constant4 : Constant  Value=Cylinder.V0_B
  Constant5 : Constant  Value=K_end
  Constant6 : Constant  Value=b_end
  Constant7 : Constant  Value=Cylinder.stroke
  Cylinder area : Gain  Gain=Cylinder.A_A
  Cylinder area1 : Gain  Gain=Cylinder.A_A
  Cylinder area2 : Gain  Gain=Cylinder.A_A
  Gain : Gain  Gain=4000
  MATLAB Function : MATLAB Function  TreatAsAtomicUnit=on
  "Piston side area " : Gain  Gain=Cylinder.A_B
  Piston side area 1 : Gain  Gain=Cylinder.A_B
  Piston side area 2 : Gain  Gain=-Cylinder.A_B
  Product : Product
  Product1 : Product
  Tanh : Trigonometry  Operator=tanh
  dx/dt1 : InportShadow  Port=4
  p1Scope : Scope
  pScope : Scope
  x1 : InportShadow  Port=3
  p : Outport
  p1 : Outport  Port=2
  F : Outport  Port=3
  wires:
  B/1 -> Chamber B/4(" B"), Chamber A/4(" B")
  Piston side area 2/1 -> Chamber B/2(" dV/dt")
  Constant/1 -> Product/1
  Add3/1 -> Chamber B/3(" V")
  x/1 -> Add4/2, Cylinder area2/1
  Chamber B/1(p) -> p1Scope/1, p1/1, "Piston side area "/1
  Tanh/1 -> Product1/2
  Q_A/1 -> Chamber A/1(Net Flow)
  Gain/1 -> Tanh/1
  Chamber A/1(p) -> pScope/1, p/1, Cylinder area/1
  Constant4/1 -> Add3/2
  Piston side area 1/1 -> Add3/1
  Add/1 -> F/1
  Q_B/1 -> Chamber B/1(Net Flow)
  dx/dt/1 -> Product/2, Gain/1, Cylinder area1/1, Piston side area 2/1
  Constant1/1 -> Product1/1
  Cylinder area2/1 -> Add2/1
  Constant2/1 -> Add2/2
  Product1/1 -> Add1/2
  Add1/1 -> Add/4
  Cylinder area1/1 -> Chamber A/2(" dV/dt")  "dV_A/dt"
  Product/1 -> Add1/1
  "Piston side area "/1 -> Add/2
  Add2/1 -> Chamber A/3(" V")  "V_A"
  Cylinder area/1 -> Add/1
  Add4/1 -> Piston side area 1/1
  Constant3/1 -> Add4/1
  dx/dt1/1 -> MATLAB Function/2(v)
  x1/1 -> MATLAB Function/1(x)
  Constant5/1 -> MATLAB Function/3(K_end)
  Constant6/1 -> MATLAB Function/4(b_end)
  MATLAB Function/1(F_end) -> Add/3
  Constant7/1 -> MATLAB Function/5(Cylinder2stroke)

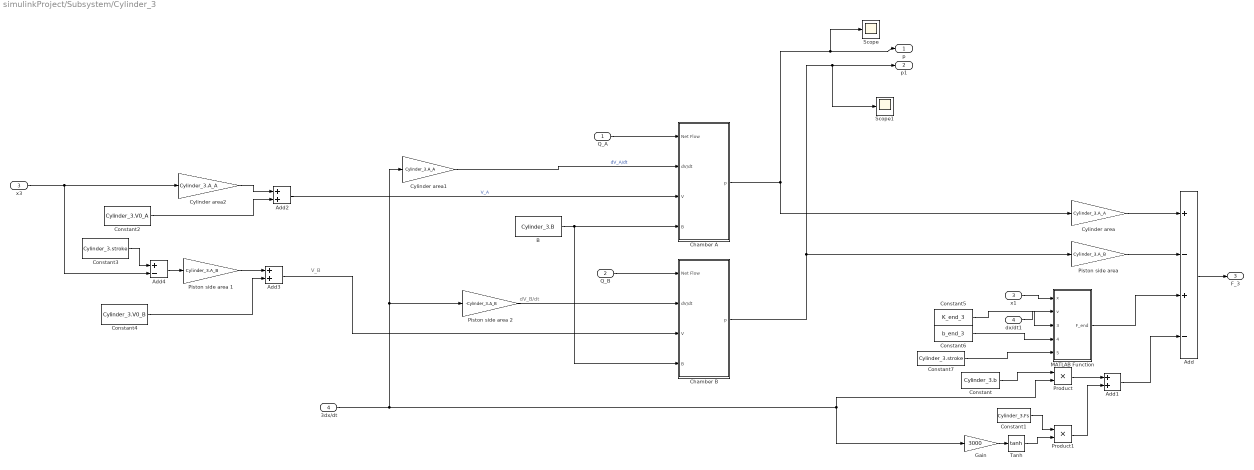
== system simulinkProject/Subsystem/Cylinder_3 ==
  note: dV_B/dt
  note: V_B
  Q_A : Inport
  Q_B : Inport  Port=2
  x3 : Inport  Port=3
  3dx/dt : Inport  Port=4
  Add : Sum  Inputs=+-+-
  Add1 : Sum
  Add2 : Sum
  Add3 : Sum
  Add4 : Sum  Inputs=+-
  B : Constant  Value=Cylinder_3.B
  Chamber A : Subsystem  mask(Hydraulic){pinitial=Cylinder_3.p0_A}
      mask prompts: pinitial "Initial pressure [Pa] :"
      mask help: Lumped fluid volume. Pressure is limited greater or equal to zero by saturation block corresponding to a rough model of cavitation.
      mask Help: eval('hydlibdoc(''vol_cav_doc'')')
  Chamber B : Subsystem  mask(Hydraulic){pinitial=Cylinder_3.p0_B}
      mask prompts: pinitial "Initial pressure [Pa] :"
      mask help: Lumped fluid volume. Pressure is limited greater or equal to zero by saturation block corresponding to a rough model of cavitation.
      mask Help: eval('hydlibdoc(''vol_cav_doc'')')
  Constant : Constant  Value=Cylinder_3.b
  Constant1 : Constant  Value=Cylinder_3.Fs
  Constant2 : Constant  Value=Cylinder_3.V0_A
  Constant3 : Constant  Value=Cylinder_3.stroke
  Constant4 : Constant  Value=Cylinder_3.V0_B
  Constant5 : Constant  Value=K_end_3
  Constant6 : Constant  Value=b_end_3
  Constant7 : Constant  Value=Cylinder_3.stroke
  Cylinder area : Gain  Gain=Cylinder_3.A_A
  Cylinder area1 : Gain  Gain=Cylinder_3.A_A
  Cylinder area2 : Gain  Gain=Cylinder_3.A_A
  Gain : Gain  Gain=3000
  MATLAB Function : MATLAB Function  TreatAsAtomicUnit=on
  "Piston side area " : Gain  Gain=Cylinder_3.A_B
  Piston side area 1 : Gain  Gain=Cylinder_3.A_B
  Piston side area 2 : Gain  Gain=-Cylinder_3.A_B
  Product : Product
  Product1 : Product
  Scope : Scope
  Scope1 : Scope
  Tanh : Trigonometry  Operator=tanh
  dx/dt1 : InportShadow  Port=4
  x1 : InportShadow  Port=3
  p : Outport
  p1 : Outport  Port=2
  F_3 : Outport  Port=3
  wires:
  B/1 -> Chamber B/4(" B"), Chamber A/4(" B")
  Piston side area 2/1 -> Chamber B/2(" dV/dt")
  Constant/1 -> Product/1
  Add3/1 -> Chamber B/3(" V")
  x3/1 -> Add4/2, Cylinder area2/1
  Tanh/1 -> Product1/2
  Q_A/1 -> Chamber A/1(Net Flow)
  Gain/1 -> Tanh/1
  Chamber A/1(p) -> Scope/1, p/1, Cylinder area/1
  Constant4/1 -> Add3/2
  Piston side area 1/1 -> Add3/1
  Add/1 -> F_3/1
  Q_B/1 -> Chamber B/1(Net Flow)
  3dx/dt/1 -> Product/2, Gain/1, Cylinder area1/1, Piston side area 2/1
  Constant1/1 -> Product1/1
  Cylinder area2/1 -> Add2/1
  Constant2/1 -> Add2/2
  Product1/1 -> Add1/2
  Cylinder area1/1 -> Chamber A/2(" dV/dt")  "dV_A/dt"
  Product/1 -> Add1/1
  "Piston side area "/1 -> Add/2
  Add2/1 -> Chamber A/3(" V")  "V_A"
  Cylinder area/1 -> Add/1
  Add4/1 -> Piston side area 1/1
  Constant3/1 -> Add4/1
  dx/dt1/1 -> MATLAB Function/2(v)
  x1/1 -> MATLAB Function/1(x)
  Constant5/1 -> MATLAB Function/3(K_end_3)
  Constant6/1 -> MATLAB Function/4(b_end_3)
  MATLAB Function/1(F_end) -> Add/3
  Add1/1 -> Add/4
  Chamber B/1(p) -> Scope1/1, p1/1, "Piston side area "/1
  Constant7/1 -> MATLAB Function/5(Cylinder3stroke)

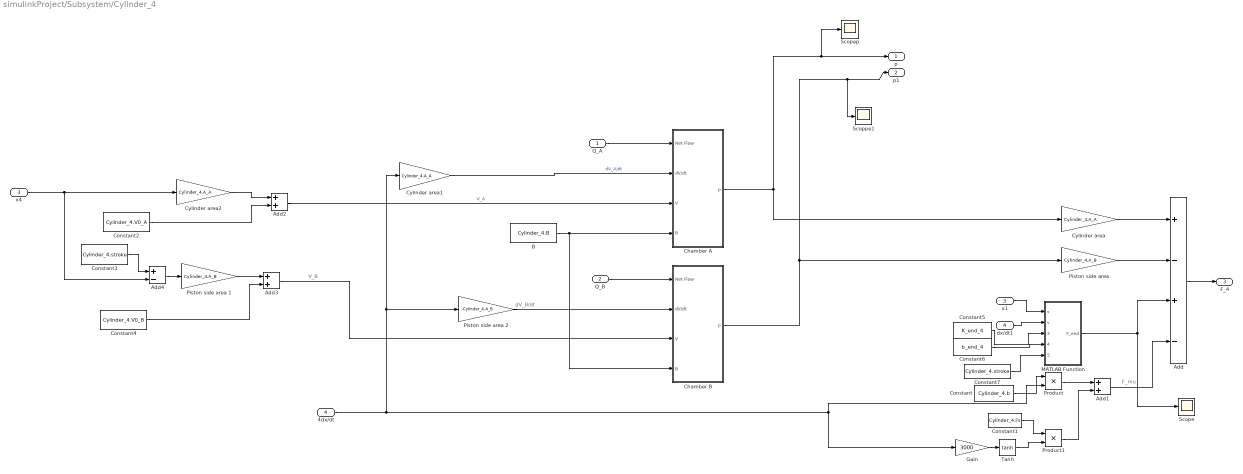
== system simulinkProject/Subsystem/Cylinder_4 ==
  note: dV_B/dt
  note: V_B
  note: F_mu
  Q_A : Inport
  Q_B : Inport  Port=2
  x4 : Inport  Port=3
  4dx/dt : Inport  Port=4
  Add : Sum  Inputs=+-+-
  Add1 : Sum
  Add2 : Sum
  Add3 : Sum
  Add4 : Sum  Inputs=+-
  B : Constant  Value=Cylinder_4.B
  Chamber A : Subsystem  mask(Hydraulic){pinitial=Cylinder_4.p0_A}
      mask prompts: pinitial "Initial pressure [Pa] :"
      mask help: Lumped fluid volume. Pressure is limited greater or equal to zero by saturation block corresponding to a rough model of cavitation.
      mask Help: eval('hydlibdoc(''vol_cav_doc'')')
  Chamber B : Subsystem  mask(Hydraulic){pinitial=Cylinder_4.p0_B}
      mask prompts: pinitial "Initial pressure [Pa] :"
      mask help: Lumped fluid volume. Pressure is limited greater or equal to zero by saturation block corresponding to a rough model of cavitation.
      mask Help: eval('hydlibdoc(''vol_cav_doc'')')
  Constant : Constant  Value=Cylinder_4.b
  Constant1 : Constant  Value=Cylinder_4.Fs
  Constant2 : Constant  Value=Cylinder_4.V0_A
  Constant3 : Constant  Value=Cylinder_4.stroke
  Constant4 : Constant  Value=Cylinder_4.V0_B
  Constant5 : Constant  Value=K_end_4
  Constant6 : Constant  Value=b_end_4
  Constant7 : Constant  Value=Cylinder_4.stroke
  Cylinder area : Gain  Gain=Cylinder_4.A_A
  Cylinder area1 : Gain  Gain=Cylinder_4.A_A
  Cylinder area2 : Gain  Gain=Cylinder_4.A_A
  Gain : Gain  Gain=3000
  MATLAB Function : MATLAB Function  TreatAsAtomicUnit=on
  "Piston side area " : Gain  Gain=Cylinder_4.A_B
  Piston side area 1 : Gain  Gain=Cylinder_4.A_B
  Piston side area 2 : Gain  Gain=-Cylinder_4.A_B
  Product : Product
  Product1 : Product
  Scope : Scope
  Scopep : Scope
  Scoppe1 : Scope
  Tanh : Trigonometry  Operator=tanh
  dx/dt1 : InportShadow  Port=4
  x1 : InportShadow  Port=3
  p : Outport
  p1 : Outport  Port=2
  F_4 : Outport  Port=3
  wires:
  B/1 -> Chamber B/4(" B"), Chamber A/4(" B")
  Piston side area 2/1 -> Chamber B/2(" dV/dt")
  Constant/1 -> Product/1
  Add3/1 -> Chamber B/3(" V")
  x4/1 -> Add4/2, Cylinder area2/1
  Chamber B/1(p) -> Scoppe1/1, p1/1, "Piston side area "/1
  Tanh/1 -> Product1/2
  Q_A/1 -> Chamber A/1(Net Flow)
  Gain/1 -> Tanh/1
  Chamber A/1(p) -> Scopep/1, p/1, Cylinder area/1
  Constant4/1 -> Add3/2
  Piston side area 1/1 -> Add3/1
  Add/1 -> F_4/1
  Q_B/1 -> Chamber B/1(Net Flow)
  4dx/dt/1 -> Product/2, Gain/1, Cylinder area1/1, Piston side area 2/1
  Constant1/1 -> Product1/1
  Cylinder area2/1 -> Add2/1
  Constant2/1 -> Add2/2
  Product1/1 -> Add1/2
  Add1/1 -> Add/4
  Cylinder area1/1 -> Chamber A/2(" dV/dt")  "dV_A/dt"
  Product/1 -> Add1/1
  "Piston side area "/1 -> Add/2
  Add2/1 -> Chamber A/3(" V")  "V_A"
  Cylinder area/1 -> Add/1
  Add4/1 -> Piston side area 1/1
  Constant3/1 -> Add4/1
  dx/dt1/1 -> MATLAB Function/2(v)
  x1/1 -> MATLAB Function/1(x)
  Constant5/1 -> MATLAB Function/3(K_end_4)
  Constant6/1 -> MATLAB Function/4(b_end_4)
  MATLAB Function/1(F_end) -> Add/3, Scope/1
  Constant7/1 -> MATLAB Function/5(Cylinder4stroke)
